simulink model "A_Linear_Sim"  (R2020a)
settings: Solver=VariableStepAuto  StartTime=0.0  StopTime=10.0  FixedStep=5e-3  RelTol=1e-3
values from neighbouring files (symbols this model uses):
  k = 10    [A_Linear.m]
  K_Linear = value(Y)/value(Q)    [A_Linear.m]
  x0 = 2    [A_Linear.m]
settings Model: Creator=FawaD KhaN  LastModifiedBy=FawaD KhaN
settings DebuggingCC: StringTruncationChecking=none

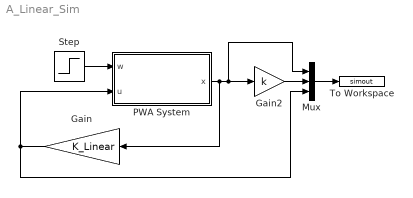
== system A_Linear_Sim ==
  Gain : Gain  Gain=K_Linear
  Gain2 : Gain  Gain=k
  Mux : Mux  Inputs=3
  PWA System : Subsystem
  Step : Step  Time=0  SampleTime=0
  To Workspace : ToWorkspace  VariableName=simout  SaveFormat=Timeseries  SampleTime=-1
  wires:
  PWA System/1(x) -> Gain/1, Mux/1, Gain2/1
  Step/1 -> PWA System/1(w)
  Gain/1 -> Mux/3, PWA System/2(u)
  Gain2/1 -> Mux/2
  Mux/1 -> To Workspace/1

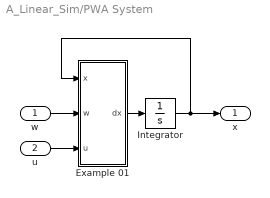
== system A_Linear_Sim/PWA System ==
  w : Inport
  u : Inport  Port=2
  Example 01 : MATLAB Function  TreatAsAtomicUnit=on
  Integrator : Integrator  InitialCondition=x0
  x : Outport
  wires:
  u/1 -> Example 01/3(u)
  Example 01/1(dx) -> Integrator/1
  Integrator/1 -> Example 01/1(x), x/1
  w/1 -> Example 01/2(w)

== matlab function A_Linear_Sim/PWA System/Example 01 ==
  data: x input; w input; u input; dx output
function dx = fcn(x,w,u)

dx = -5*x*(1+(sin(x))^2) + w + u;

end
